simulink model "robot_hardware_equipment"  (R2024b)
settings: Solver=VariableStepAuto  StartTime=0.0  StopTime=10.0  RelTol=1e-3
values from neighbouring files (symbols this model uses):
  Fv11 = 2 * ( gbox.B + wheel.B )    [MATRIX.m]
  g = 9.81    [balrob_params.m]
  g1 = 0    [MATRIX.m]
  M11 = 2 * wheel.Iyy + 2 * gbox.N^2 * mot.rot.Iyy + ( body.m + 2 * wheel.m + 2 * mot.rot.m ) * wheel.r^2    [MATRIX.m]
  M22 = body.Iyy + 2 * ( 1 - gbox.N )^2 * mot.rot.Iyy + body.m * body.zb^2 + 2 * mot.rot.m * mot.rot.zb^2    [MATRIX.m]
  ms22g = 1/g    (= 0.101936799185)    [balrob_params.m]
  Ts = 1e-2    (= 0.01)    [balrob_params.m]
  ua2tau1 = ( 2 * gbox.N * mot.Kt / mot.R) * [1, -1]'    [MATRIX.m]
undefined symbols (not defined in the file or in its folder): body, drv, gbox, mot, sens, wheel
settings Model: Creator=apple  LastModifiedBy=Davide Pillon

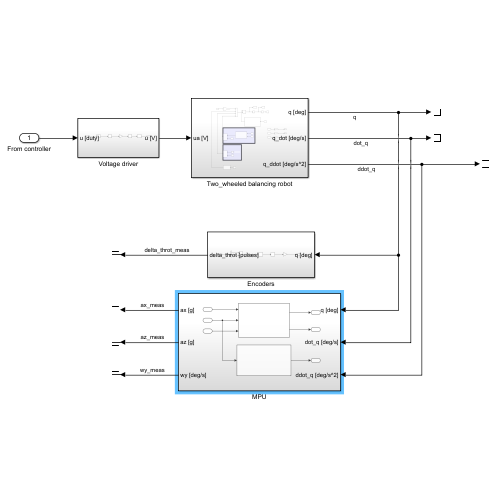
[thumbnail: Simulink's stored preview of the top-level diagram]
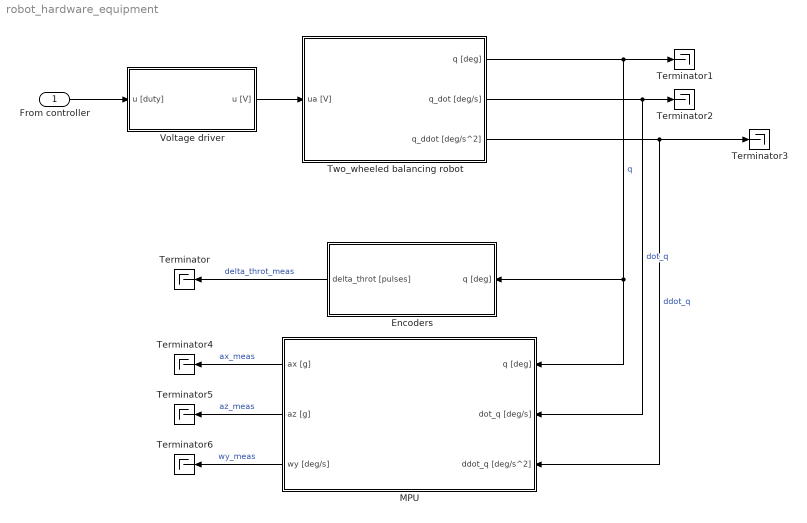
== system robot_hardware_equipment ==
  From controller : Inport
  Encoders : Subsystem
  MPU : Subsystem
  Terminator{,1..6} (7 alike) : Terminator
  Two_wheeled balancing robot : Subsystem
  Voltage driver : Subsystem
  wires:
  MPU/1(ax [g]) -> Terminator4/1  "ax_meas"
  MPU/2(az [g]) -> Terminator5/1  "az_meas"
  MPU/3(wy [deg/s]) -> Terminator6/1  "wy_meas"
  Two_wheeled balancing robot/1(q [deg]) -> Terminator1/1, MPU/1(q [deg]), Encoders/1(q [deg])  "q"
  Two_wheeled balancing robot/2(q_dot [deg/s]) -> Terminator2/1, MPU/2(dot_q [deg/s])  "dot_q"
  Two_wheeled balancing robot/3(q_ddot [deg/s^2]) -> MPU/3(ddot_q [deg/s^2]), Terminator3/1  "ddot_q"
  Encoders/1(delta_throt [pulses]) -> Terminator/1  "delta_throt_meas"
  From controller/1 -> Voltage driver/1(u [duty])
  Voltage driver/1(u [V]) -> Two_wheeled balancing robot/1("ua [V] ")

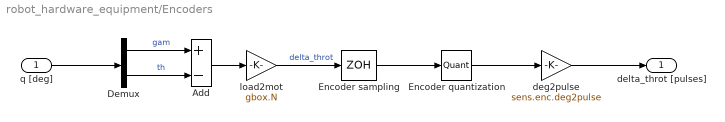
== system robot_hardware_equipment/Encoders ==
  q [deg] : Inport
  Add : Sum  Inputs=+-
  Demux : Demux  Outputs=2
  Encoder quantization : Quantizer  QuantizationInterval=sens.enc.pulse2deg
  Encoder sampling : ZeroOrderHold  SampleTime=Ts
  deg2pulse : Gain  Gain=sens.enc.deg2pulse
  load2mot : Gain  Gain=gbox.N
  delta_throt [pulses] : Outport
  wires:
  Encoder quantization/1 -> deg2pulse/1
  Encoder sampling/1 -> Encoder quantization/1
  Demux/2 -> Add/2  "th"
  q [deg]/1 -> Demux/1
  Demux/1 -> Add/1  "gam"
  load2mot/1 -> Encoder sampling/1  "delta_throt"
  Add/1 -> load2mot/1
  deg2pulse/1 -> delta_throt [pulses]/1

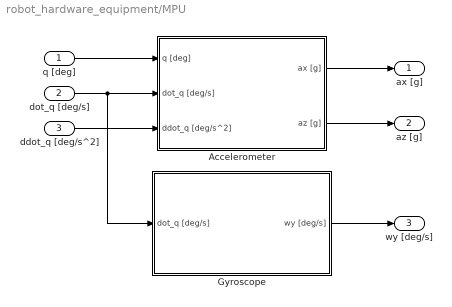
== system robot_hardware_equipment/MPU ==
  q [deg] : Inport
  dot_q [deg/s] : Inport  Port=2
  ddot_q [deg/s^2] : Inport  Port=3
  Accelerometer : Subsystem
  Gyroscope : Subsystem
  ax [g] : Outport
  az [g] : Outport  Port=2
  wy [deg/s] : Outport  Port=3
  wires:
  Gyroscope/1(wy [deg/s]) -> wy [deg/s]/1
  Accelerometer/1(ax [g]) -> ax [g]/1
  ddot_q [deg/s^2]/1 -> Accelerometer/3(ddot_q [deg/s^2])
  q [deg]/1 -> Accelerometer/1(q [deg])
  Accelerometer/2(az [g]) -> az [g]/1
  dot_q [deg/s]/1 -> Accelerometer/2(dot_q [deg/s]), Gyroscope/1(dot_q [deg/s])

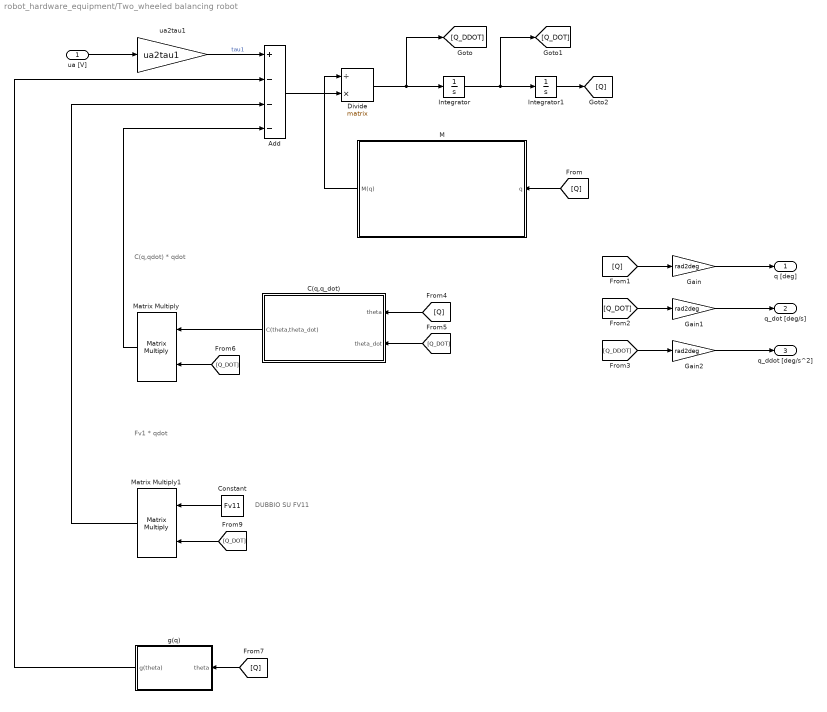
== system robot_hardware_equipment/Two_wheeled balancing robot ==
  note: DUBBIO SU FV11
  note: C(q,qdot) * qdot
  note: Fv1 * qdot
  "ua [V] " : Inport
  Add : Sum  Inputs=+---
  C(q,q_dot) : Subsystem
  Constant : Constant  Value=Fv11
  Divide : Product  Inputs=/*  Multiplication=Matrix(*)
  Gain : Gain  Gain=rad2deg
  Gain1 : Gain  Gain=rad2deg
  Gain2 : Gain  Gain=rad2deg
  Integrator : Integrator
  Integrator1 : Integrator
  M : Subsystem
  Matrix Multiply : Product  Multiplication=Matrix(*)
  Matrix Multiply1 : Product  Multiplication=Matrix(*)
  g(q) : Subsystem
  ua2tau1 : Gain  Gain=ua2tau1
  q [deg] : Outport
  q_dot [deg/s] : Outport  Port=2
  q_ddot [deg/s^2] : Outport  Port=3
  wires:
  [Q_DOT] -> Matrix Multiply1/2
  [Q] -> M/1(q)
  Divide/1 -> [Q_DDOT], Integrator/1
  Matrix Multiply/1 -> Add/4
  Gain/1 -> q [deg]/1
  [Q_DOT] -> Matrix Multiply/2
  g(q)/1(g(theta)) -> Add/2
  [Q_DOT] -> C(q,q_dot)/2(theta_dot)
  ua2tau1/1 -> Add/1  "tau1"
  [Q_DOT] -> Gain1/1
  Constant/1 -> Matrix Multiply1/1
  Integrator1/1 -> [Q]
  Integrator/1 -> [Q_DOT], Integrator1/1
  [Q] -> Gain/1
  [Q] -> C(q,q_dot)/1(theta)
  "ua [V] "/1 -> ua2tau1/1
  Add/1 -> Divide/2
  Matrix Multiply1/1 -> Add/3
  [Q_DDOT] -> Gain2/1
  Gain2/1 -> q_ddot [deg/s^2]/1
  M/1(M(q)) -> Divide/1
  [Q] -> g(q)/1(theta)
  C(q,q_dot)/1(C(theta,theta_dot)) -> Matrix Multiply/1
  Gain1/1 -> q_dot [deg/s]/1

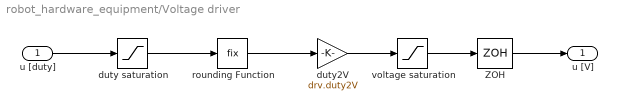
== system robot_hardware_equipment/Voltage driver ==
  u [duty] : Inport
  ZOH : ZeroOrderHold  SampleTime=Ts
  duty saturation : Saturate  UpperLimit=drv.dutymax  LowerLimit=-drv.dutymax
  duty2V : Gain  Gain=drv.duty2V
  rounding Function : Rounding  Operator=fix
  voltage saturation : Saturate  UpperLimit=drv.Vbus  LowerLimit=-drv.Vbus
  u [V] : Outport
  wires:
  duty saturation/1 -> rounding Function/1
  u [duty]/1 -> duty saturation/1
  rounding Function/1 -> duty2V/1
  voltage saturation/1 -> ZOH/1
  ZOH/1 -> u [V]/1
  duty2V/1 -> voltage saturation/1

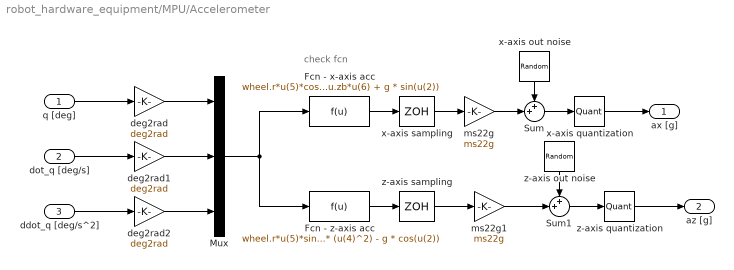
== system robot_hardware_equipment/MPU/Accelerometer ==
  note: check fcn
  q [deg] : Inport
  dot_q [deg/s] : Inport  Port=2
  ddot_q [deg/s^2] : Inport  Port=3
  Fcn - x-axis acc : Fcn  Expr=wheel.r*u(5)*cos(u(2)) + sens.mpu.zb*u(6) + g * sin(u(2))
  Fcn - z-axis acc : Fcn  Expr=wheel.r*u(5)*sin(u(2)) - sens.mpu.zb * (u(4)^2) - g * cos(u(2))
  Mux : Mux  Inputs=3
  Sum : Sum  Inputs=++|
  Sum1 : Sum  Inputs=++|
  deg2rad : Gain  Gain=deg2rad
  deg2rad1 : Gain  Gain=deg2rad
  deg2rad2 : Gain  Gain=deg2rad
  ms22g : Gain  Gain=ms22g
  ms22g1 : Gain  Gain=ms22g
  x-axis out noise : RandomNumber  Variance=sens.mpu.acc.noisevar  SampleTime=Ts
  x-axis quantization : Quantizer  QuantizationInterval=sens.mpu.acc.LSB2g
  x-axis sampling : ZeroOrderHold  SampleTime=Ts
  z-axis out noise : RandomNumber  Variance=sens.mpu.acc.noisevar  SampleTime=Ts
  z-axis quantization : Quantizer  QuantizationInterval=sens.mpu.acc.LSB2g
  z-axis sampling : ZeroOrderHold  SampleTime=Ts
  ax [g] : Outport
  az [g] : Outport  Port=2
  wires:
  x-axis quantization/1 -> ax [g]/1
  Fcn - z-axis acc/1 -> z-axis sampling/1
  dot_q [deg/s]/1 -> deg2rad1/1
  q [deg]/1 -> deg2rad/1
  Fcn - x-axis acc/1 -> x-axis sampling/1
  ddot_q [deg/s^2]/1 -> deg2rad2/1
  Mux/1 -> Fcn - z-axis acc/1, Fcn - x-axis acc/1
  z-axis quantization/1 -> az [g]/1
  z-axis out noise/1 -> Sum1/1
  z-axis sampling/1 -> ms22g1/1
  deg2rad1/1 -> Mux/2
  ms22g/1 -> Sum/2
  ms22g1/1 -> Sum1/2
  x-axis out noise/1 -> Sum/1
  Sum1/1 -> z-axis quantization/1
  deg2rad/1 -> Mux/1
  deg2rad2/1 -> Mux/3
  x-axis sampling/1 -> ms22g/1
  Sum/1 -> x-axis quantization/1

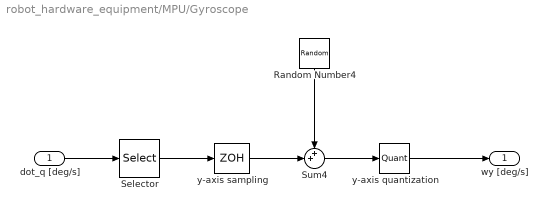
== system robot_hardware_equipment/MPU/Gyroscope ==
  dot_q [deg/s] : Inport
  "Random Number4 " : RandomNumber  Variance=sens.mpu.gyro.noisevar  SampleTime=Ts
  "Selector " : Selector  InputPortWidth=2  IndexOptions=Index vector (dialog)  Indices=2  OutputSizes=1
  "Sum4 " : Sum  Inputs=++|
  y-axis quantization : Quantizer  QuantizationInterval=sens.mpu.gyro.LSB2degs
  y-axis sampling : ZeroOrderHold  SampleTime=Ts
  wy [deg/s] : Outport
  wires:
  "Random Number4 "/1 -> "Sum4 "/1
  y-axis sampling/1 -> "Sum4 "/2
  "Sum4 "/1 -> y-axis quantization/1
  y-axis quantization/1 -> wy [deg/s]/1
  dot_q [deg/s]/1 -> "Selector "/1
  "Selector "/1 -> y-axis sampling/1

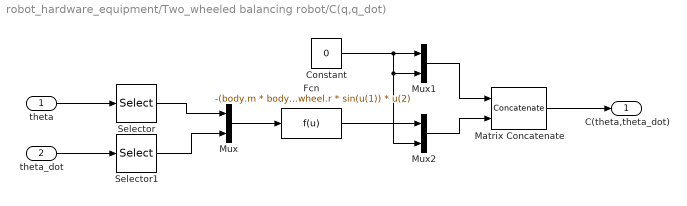
== system robot_hardware_equipment/Two_wheeled balancing robot/C(q,q_dot) ==
  theta : Inport
  theta_dot : Inport  Port=2
  Constant : Constant  Value=0
  Fcn : Fcn  Expr=-(body.m * body.zb + 2 * mot.rot.m * mot.rot.zb ) * wheel.r * sin(u(1)) * u(2)
  Matrix Concatenate : Concatenate  Mode=Multidimensional array  ConcatenateDimension=2
  Mux : Mux  Inputs=2
  Mux1 : Mux  Inputs=2
  Mux2 : Mux  Inputs=2
  Selector : Selector  InputPortWidth=2  IndexOptions=Index vector (dialog)  Indices=[2]  OutputSizes=1
  Selector1 : Selector  InputPortWidth=2  IndexOptions=Index vector (dialog)  Indices=[2]  OutputSizes=1
  C(theta,theta_dot) : Outport
  wires:
  Matrix Concatenate/1 -> C(theta,theta_dot)/1
  Mux2/1 -> Matrix Concatenate/2
  theta/1 -> Selector/1
  Constant/1 -> Mux2/2, Mux1/2, Mux1/1
  Mux/1 -> Fcn/1
  Mux1/1 -> Matrix Concatenate/1
  Selector1/1 -> Mux/2
  theta_dot/1 -> Selector1/1
  Selector/1 -> Mux/1
  Fcn/1 -> Mux2/1

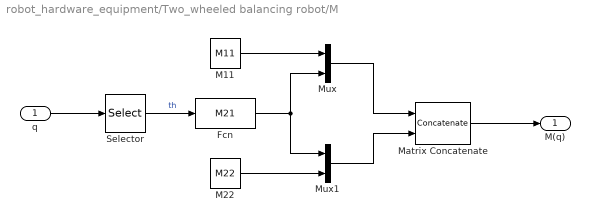
== system robot_hardware_equipment/Two_wheeled balancing robot/M ==
  q : Inport
  Fcn : Fcn  Expr=M21
  M11 : Constant  Value=M11
  M22 : Constant  Value=M22
  Matrix Concatenate : Concatenate  Mode=Multidimensional array  ConcatenateDimension=2
  Mux : Mux  Inputs=2
  Mux1 : Mux  Inputs=2
  Selector : Selector  InputPortWidth=2  IndexOptions=Index vector (dialog)  Indices=[2]  OutputSizes=1
  M(q) : Outport
  wires:
  Matrix Concatenate/1 -> M(q)/1
  M22/1 -> Mux1/2
  Fcn/1 -> Mux1/1, Mux/2
  q/1 -> Selector/1
  Mux/1 -> Matrix Concatenate/1
  Mux1/1 -> Matrix Concatenate/2
  Selector/1 -> Fcn/1  "th"
  M11/1 -> Mux/1

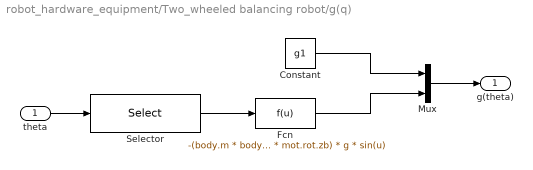
== system robot_hardware_equipment/Two_wheeled balancing robot/g(q) ==
  theta : Inport
  Constant : Constant  Value=g1
  Fcn : Fcn  Expr=-(body.m * body.zb + 2 * mot.rot.m * mot.rot.zb) * g * sin(u)
  Mux : Mux  Inputs=2
  Selector : Selector  InputPortWidth=2  IndexOptions=Index vector (dialog)  Indices=[2]  OutputSizes=1
  g(theta) : Outport
  wires:
  Constant/1 -> Mux/1
  Fcn/1 -> Mux/2
  Selector/1 -> Fcn/1
  theta/1 -> Selector/1
  Mux/1 -> g(theta)/1
